simulink model "Channelizer_kernel"  (R2024a)
settings: Solver=VariableStepAuto  StartTime=0.0  StopTime=inf  RelTol=1e-3
InitFcn:
  | init
  | init_kernel
values from neighbouring files (symbols this model uses):
  N = 2*1024    (= 2048)    [hil.m]    (also in init.m = 256)
undefined symbols (not defined in the file or in its folder): ch0, ch1, ch10, ch11, ch12, ch13, ch14, ch15, ch2, ch3, ch4, ch5, ch6, ch7, ch8, ch9, S, vsva2197, xcvc1902
libraries: aieBasic x56, aieUtilities x39, hlsBasic x3, dspindex x2, vmcUtilities x1, commchan3 x1, commrflib2 x1, commfilt2 x1, commrandsrc3 x1, commdigbbndam3 x1
(part 2 of 3)

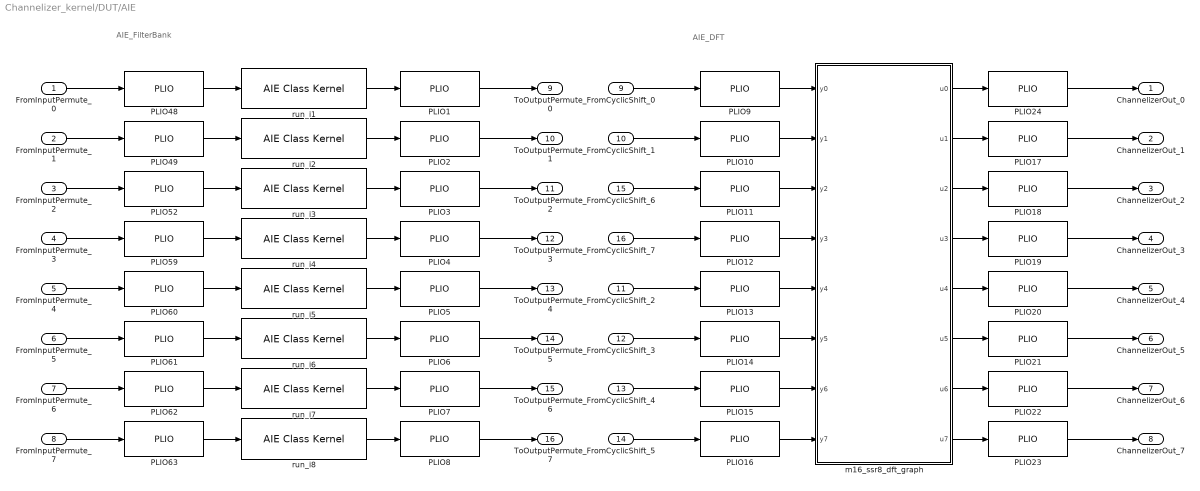
== system Channelizer_kernel/DUT/AIE ==
  note: AIE_DFT
  note: AIE_FilterBank
  FromInputPermute_0 : Inport
  FromInputPermute_1 : Inport  Port=2
  FromInputPermute_2 : Inport  Port=3
  FromInputPermute_3 : Inport  Port=4
  FromInputPermute_4 : Inport  Port=5
  FromInputPermute_5 : Inport  Port=6
  FromInputPermute_6 : Inport  Port=7
  FromInputPermute_7 : Inport  Port=8
  FromCyclicShift_0 : Inport  Port=9
  FromCyclicShift_1 : Inport  Port=10
  FromCyclicShift_2 : Inport  Port=11
  FromCyclicShift_3 : Inport  Port=12
  FromCyclicShift_4 : Inport  Port=13
  FromCyclicShift_5 : Inport  Port=14
  FromCyclicShift_6 : Inport  Port=15
  FromCyclicShift_7 : Inport  Port=16
  PLIO{1..24,48..49,52,59..63} (32 alike) : aieBasic/PLIO  PlioWidth=64  PlioFreqSpec=on  PlioFreq=625  ColLocation=0  channel=0  blockJsonConstraints=[]  deprecateConstraints=0
  m16_ssr8_dft_graph : Subsystem
  run_i1 : aieBasic/AIE Class Kernel  KernelAllAttrs=|  PortNames={'sig_i'; 'sig_o'}  PortSerializedTypes={'{Q2{P{Tinput_stream{1{t{Scint16}}}}}}'; '{Q2{P{Toutput_stream{1{t{Scint16}}}}}}'}  PortWindowSizes={0.000000000000000000e+00; 0.000000000000000000e+00}  PortWindowMargins={0.000000000000000000e+00; 0.000000000000000000e+00}  PortSynchronicities={'auto', 'auto'}  PortSignalSizes={0.000000000000000000e+00; 8.192000000000000000e+03}  ClassTemplateSpecKind=implicit  ClassTemplateParamNames={'pattern'; 'NSAMP'}  ClassTemplateParamKinds={'nontype'; 'nontype'}  ClassTemplateParamTypes={'unsigned int'; 'unsigned int'}  ClassTemplateParamValues={'0', '8192'}  ClassCtorParamNames={'taps0_i'; 'taps1_i'}  ClassCtorParamSerializedTypes={'{R{C{Bi16}64}}'; '{R{C{Bi16}64}}'}  ClassCtorParamValues={'[0;2;-4;6;-13;54;-178;1985;-20;88;-287;1822;-22;100;-326;1570;2042;6;-4;2;259;-80;23;-8;569;-166;49;-9;911;-248;74;-14;-19;93;-307;1256;-14;74;-248;911;-9;49;-166;569;-8;23;-80;259;1256;-307;93;-19;1570;-326;100;-22;1822;-287;88;-20;1985;-178;54;-13]', '[6;12;-40;124;-6;28;-95;2027;-17;74;-241;1916;-22;97;-314;1706;2027;-95;28;-6;124;-40;12;6;408;-123;36;-8;737;-209;62;-12;-21;99;-322;1419;-17;85;-281;1085;-12;62;-209;737;-8;36;-123;408;1085;-281;85;-17;1419;-322;99;-21;1706;-314;97;-22;1916;-241;74;-17]'}  ClassIndex=1  ClassCtorIndex=1  ClassTabVisible=on  ClassTemplateParamsVisible=on  ClassCtorDeclVisible=on  ClassCtorParamsVisible=on  FunctionTabVisible=on  FunctionDecl=|  PortAttrs={ 'input', 'sig_i', 'input_stream_cint16 * restrict', '', '', '', ''; 'output', 'sig_o', 'output_stream_cint16 * restrict', '', '', '', '4*N' }  PortAttrsEnables={'off', 'off', 'off', 'off', 'off', 'off', 'off';'off', 'off', 'off', 'off', 'off', 'off', 'on'}  SampleTime=-1  ClassDeclTypeOptions=C[1 1]@t74@template < unsigned int pattern, unsigned int NSAMP > class polyphase_fir;  ClassDecl=template < unsigned int pattern, unsigned int NSAMP > class polyphase_fir;  ClassTemplateParams={ 'pattern', 'unsigned int', '0'; 'NSAMP', 'unsigned int', '4*N' }  ClassTemplateParamsEnables={'off', 'off', 'on';'off', 'off', 'on'}  ClassCtorDeclTypeOptions=C[1 1]@t69@polyphase_fir(int16 ( & taps0_i ) [ 64 ], int16 ( & taps1_i ) [ 64 ])  ClassCtorDecl=polyphase_fir(int16 ( & taps0_i ) [ 64 ], int16 ( & taps1_i ) [ 64 ])  ClassCtorParams={ 'taps0_i', 'int16 ( &) [ 64 ]', 'tile0_tapsA'; 'taps1_i', 'int16 ( &) [ 64 ]', 'tile0_tapsB' }  KernelHeaderFile=aie/polyphase_fir.h  KernelClassName=polyphase_fir  KernelFunction=run_i  KernelSourceFile=aie/polyphase_fir.cpp  KernelSearchPaths={}  PreProcOptions={}  blockJsonConstraints=[]
      KernelAllAttrs=|
      | s[12;12;9;9;19;14;21;23;21;23;24;21;15;17;12;24;26;26;26;27;28;9;21;23;23;23;24;25;14;19;19;29]@FunctionNameDeclFileNamePortNamesPortTypesPortSerializedTypesPortDirectionsPortWindowSizeEnablesPortWindowMarginEnablesPortBufferSizeEnablesPortBufferMarginEnablesPortSynchronicityEnablesPortSignalSizeEnablesPortBufferSizesPortBufferMarginsFunctionDeclFunctionTemplateSpecKindFunctionTemplateParamNamesFunctionTemplateParamKindsFunctionTemplateParamTypesFunctionTemplateParamValuesFunctionTemplateParamEnablesClassDeclClassTemplateSpecKindClassTemplateParamNamesClassTemplateParamKindsClassTemplateParamTypesClassTemplateParamValuesClassTemplateParamEnablesClassCtorDeclsClassCtorParamNamesClassCtorParamTypesClassCtorParamSerializedTypes[1 1]@C[32 1]@t5@run_it25@../../aie/polyphase_fir.hC[2 1]@t5@sig_it5@sig_oC[2 1]@t30@input_stream_cint16 * restrictt31@output_stream_cint16 * restrictC[2 1]@t37@{Q2{P{Tinput_stream{1{t{Scint16}}}}}}t38@{Q2{P{Toutput_stream{1{t{Scint16}}}}}}C[2 1]@t5@inputt6@outputC[2 1]@l0@l0@C[2 1]@l0@l0@C[2 1]@l0@l0@C[2 1]@l0@l0@C[2 1]@l0@l0@C[2 1]@l0@l1@C[2 1]@nnC[2 1]@nnt158@template < unsigned int pattern, unsigned int NSAMP > 
      | void polyphase_fir::
      | run_i(input_stream_cint16 * restrict sig_i, output_stream_cint16 * restrict sig_o)t4@nonee[0 1]@e[0 1]@e[0 1]@e[0 1]@e[0 1]@t74@template < unsigned int pattern, unsigned int NSAMP > class polyphase_fir;t8@implicitC[2 1]@t7@patternt5@NSAMPC[2 1]@t7@nontypet7@nontypeC[2 1]@t12@unsigned intt12@unsigned intC[2 1]@nnC[2 1]@l1@l1@C[1 1]@t69@polyphase_fir(int16 ( & taps0_i ) [ 64 ], int16 ( & taps1_i ) [ 64 ])C[1 1]@C[2 1]@t7@taps0_it7@taps1_iC[1 1]@C[2 1]@t17@int16 ( &) [ 64 ]t17@int16 ( &) [ 64 ]C[1 1]@C[2 1]@t14@{R{C{Bi16}64}}t14@{R{C{Bi16}64}}
      FunctionDecl=|
      | template < unsigned int pattern, unsigned int NSAMP > 
      | void polyphase_fir::
      | run_i(input_stream_cint16 * restrict sig_i, output_stream_cint16 * restrict sig_o)
  run_i2 : aieBasic/AIE Class Kernel  KernelAllAttrs=|  PortNames={'sig_i'; 'sig_o'}  PortSerializedTypes={'{Q2{P{Tinput_stream{1{t{Scint16}}}}}}'; '{Q2{P{Toutput_stream{1{t{Scint16}}}}}}'}  PortWindowSizes={0.000000000000000000e+00; 0.000000000000000000e+00}  PortWindowMargins={0.000000000000000000e+00; 0.000000000000000000e+00}  PortSynchronicities={'auto', 'auto'}  PortSignalSizes={0.000000000000000000e+00; 8.192000000000000000e+03}  ClassTemplateSpecKind=implicit  ClassTemplateParamNames={'pattern'; 'NSAMP'}  ClassTemplateParamKinds={'nontype'; 'nontype'}  ClassTemplateParamTypes={'unsigned int'; 'unsigned int'}  ClassTemplateParamValues={'1', '8192'}  ClassCtorParamNames={'taps0_i'; 'taps1_i'}  ClassCtorParamSerializedTypes={'{R{C{Bi16}64}}'; '{R{C{Bi16}64}}'}  ClassCtorParamValues={'[-8;23;-80;259;0;2;-4;6;-13;54;-178;1985;-20;88;-287;1822;1985;-178;54;-13;2042;6;-4;2;259;-80;23;-8;569;-166;49;-9;-22;100;-326;1570;-19;93;-307;1256;-14;74;-248;911;-9;49;-166;569;911;-248;74;-14;1256;-307;93;-19;1570;-326;100;-22;1822;-287;88;-20]', '[-8;36;-123;408;6;12;-40;124;-6;28;-95;2027;-17;74;-241;1916;1916;-241;74;-17;2027;-95;28;-6;124;-40;12;6;408;-123;36;-8;-22;97;-314;1706;-21;99;-322;1419;-17;85;-281;1085;-12;62;-209;737;737;-209;62;-12;1085;-281;85;-17;1419;-322;99;-21;1706;-314;97;-22]'}  ClassIndex=1  ClassCtorIndex=1  ClassTabVisible=on  ClassTemplateParamsVisible=on  ClassCtorDeclVisible=on  ClassCtorParamsVisible=on  FunctionTabVisible=on  FunctionDecl=|  PortAttrs={ 'input', 'sig_i', 'input_stream_cint16 * restrict', '', '', '', ''; 'output', 'sig_o', 'output_stream_cint16 * restrict', '', '', '', '4*N' }  PortAttrsEnables={'off', 'off', 'off', 'off', 'off', 'off', 'off';'off', 'off', 'off', 'off', 'off', 'off', 'on'}  SampleTime=-1  ClassDeclTypeOptions=C[1 1]@t74@template < unsigned int pattern, unsigned int NSAMP > class polyphase_fir;  ClassDecl=template < unsigned int pattern, unsigned int NSAMP > class polyphase_fir;  ClassTemplateParams={ 'pattern', 'unsigned int', '1'; 'NSAMP', 'unsigned int', '4*N' }  ClassTemplateParamsEnables={'off', 'off', 'on';'off', 'off', 'on'}  ClassCtorDeclTypeOptions=C[1 1]@t69@polyphase_fir(int16 ( & taps0_i ) [ 64 ], int16 ( & taps1_i ) [ 64 ])  ClassCtorDecl=polyphase_fir(int16 ( & taps0_i ) [ 64 ], int16 ( & taps1_i ) [ 64 ])  ClassCtorParams={ 'taps0_i', 'int16 ( &) [ 64 ]', 'tile1_tapsA'; 'taps1_i', 'int16 ( &) [ 64 ]', 'tile1_tapsB' }  KernelHeaderFile=aie/polyphase_fir.h  KernelClassName=polyphase_fir  KernelFunction=run_i  KernelSourceFile=aie/polyphase_fir.cpp  KernelSearchPaths={}  PreProcOptions={}  blockJsonConstraints=[]
      KernelAllAttrs=|
      | s[12;12;9;9;19;14;21;23;21;23;24;21;15;17;12;24;26;26;26;27;28;9;21;23;23;23;24;25;14;19;19;29]@FunctionNameDeclFileNamePortNamesPortTypesPortSerializedTypesPortDirectionsPortWindowSizeEnablesPortWindowMarginEnablesPortBufferSizeEnablesPortBufferMarginEnablesPortSynchronicityEnablesPortSignalSizeEnablesPortBufferSizesPortBufferMarginsFunctionDeclFunctionTemplateSpecKindFunctionTemplateParamNamesFunctionTemplateParamKindsFunctionTemplateParamTypesFunctionTemplateParamValuesFunctionTemplateParamEnablesClassDeclClassTemplateSpecKindClassTemplateParamNamesClassTemplateParamKindsClassTemplateParamTypesClassTemplateParamValuesClassTemplateParamEnablesClassCtorDeclsClassCtorParamNamesClassCtorParamTypesClassCtorParamSerializedTypes[1 1]@C[32 1]@t5@run_it25@../../aie/polyphase_fir.hC[2 1]@t5@sig_it5@sig_oC[2 1]@t30@input_stream_cint16 * restrictt31@output_stream_cint16 * restrictC[2 1]@t37@{Q2{P{Tinput_stream{1{t{Scint16}}}}}}t38@{Q2{P{Toutput_stream{1{t{Scint16}}}}}}C[2 1]@t5@inputt6@outputC[2 1]@l0@l0@C[2 1]@l0@l0@C[2 1]@l0@l0@C[2 1]@l0@l0@C[2 1]@l0@l0@C[2 1]@l0@l1@C[2 1]@nnC[2 1]@nnt158@template < unsigned int pattern, unsigned int NSAMP > 
      | void polyphase_fir::
      | run_i(input_stream_cint16 * restrict sig_i, output_stream_cint16 * restrict sig_o)t4@nonee[0 1]@e[0 1]@e[0 1]@e[0 1]@e[0 1]@t74@template < unsigned int pattern, unsigned int NSAMP > class polyphase_fir;t8@implicitC[2 1]@t7@patternt5@NSAMPC[2 1]@t7@nontypet7@nontypeC[2 1]@t12@unsigned intt12@unsigned intC[2 1]@nnC[2 1]@l1@l1@C[1 1]@t69@polyphase_fir(int16 ( & taps0_i ) [ 64 ], int16 ( & taps1_i ) [ 64 ])C[1 1]@C[2 1]@t7@taps0_it7@taps1_iC[1 1]@C[2 1]@t17@int16 ( &) [ 64 ]t17@int16 ( &) [ 64 ]C[1 1]@C[2 1]@t14@{R{C{Bi16}64}}t14@{R{C{Bi16}64}}
      FunctionDecl=|
      | template < unsigned int pattern, unsigned int NSAMP > 
      | void polyphase_fir::
      | run_i(input_stream_cint16 * restrict sig_i, output_stream_cint16 * restrict sig_o)
  run_i3 : aieBasic/AIE Class Kernel  KernelAllAttrs=|  PortNames={'sig_i'; 'sig_o'}  PortSerializedTypes={'{Q2{P{Tinput_stream{1{t{Scint16}}}}}}'; '{Q2{P{Toutput_stream{1{t{Scint16}}}}}}'}  PortWindowSizes={0.000000000000000000e+00; 0.000000000000000000e+00}  PortWindowMargins={0.000000000000000000e+00; 0.000000000000000000e+00}  PortSynchronicities={'auto', 'auto'}  PortSignalSizes={0.000000000000000000e+00; 8.192000000000000000e+03}  ClassTemplateSpecKind=implicit  ClassTemplateParamNames={'pattern'; 'NSAMP'}  ClassTemplateParamKinds={'nontype'; 'nontype'}  ClassTemplateParamTypes={'unsigned int'; 'unsigned int'}  ClassTemplateParamValues={'2', '8192'}  ClassCtorParamNames={'taps0_i'; 'taps1_i'}  ClassCtorParamSerializedTypes={'{R{C{Bi16}64}}'; '{R{C{Bi16}64}}'}  ClassCtorParamValues={'[-9;49;-166;569;-8;23;-80;259;0;2;-4;6;-13;54;-178;1985;1822;-287;88;-20;1985;-178;54;-13;2042;6;-4;2;259;-80;23;-8;-20;88;-287;1822;-22;100;-326;1570;-19;93;-307;1256;-14;74;-248;911;569;-166;49;-9;911;-248;74;-14;1256;-307;93;-19;1570;-326;100;-22]', '[-12;62;-209;737;-8;36;-123;408;6;12;-40;124;-6;28;-95;2027;1706;-314;97;-22;1916;-241;74;-17;2027;-95;28;-6;124;-40;12;6;-17;74;-241;1916;-22;97;-314;1706;-21;99;-322;1419;-17;85;-281;1085;408;-123;36;-8;737;-209;62;-12;1085;-281;85;-17;1419;-322;99;-21]'}  ClassIndex=1  ClassCtorIndex=1  ClassTabVisible=on  ClassTemplateParamsVisible=on  ClassCtorDeclVisible=on  ClassCtorParamsVisible=on  FunctionTabVisible=on  FunctionDecl=|  PortAttrs={ 'input', 'sig_i', 'input_stream_cint16 * restrict', '', '', '', ''; 'output', 'sig_o', 'output_stream_cint16 * restrict', '', '', '', '4*N' }  PortAttrsEnables={'off', 'off', 'off', 'off', 'off', 'off', 'off';'off', 'off', 'off', 'off', 'off', 'off', 'on'}  SampleTime=-1  ClassDeclTypeOptions=C[1 1]@t74@template < unsigned int pattern, unsigned int NSAMP > class polyphase_fir;  ClassDecl=template < unsigned int pattern, unsigned int NSAMP > class polyphase_fir;  ClassTemplateParams={ 'pattern', 'unsigned int', '2'; 'NSAMP', 'unsigned int', '4*N' }  ClassTemplateParamsEnables={'off', 'off', 'on';'off', 'off', 'on'}  ClassCtorDeclTypeOptions=C[1 1]@t69@polyphase_fir(int16 ( & taps0_i ) [ 64 ], int16 ( & taps1_i ) [ 64 ])  ClassCtorDecl=polyphase_fir(int16 ( & taps0_i ) [ 64 ], int16 ( & taps1_i ) [ 64 ])  ClassCtorParams={ 'taps0_i', 'int16 ( &) [ 64 ]', 'tile2_tapsA'; 'taps1_i', 'int16 ( &) [ 64 ]', 'tile2_tapsB' }  KernelHeaderFile=aie/polyphase_fir.h  KernelClassName=polyphase_fir  KernelFunction=run_i  KernelSourceFile=aie/polyphase_fir.cpp  KernelSearchPaths={}  PreProcOptions={}  blockJsonConstraints=[]
      KernelAllAttrs=|
      | s[12;12;9;9;19;14;21;23;21;23;24;21;15;17;12;24;26;26;26;27;28;9;21;23;23;23;24;25;14;19;19;29]@FunctionNameDeclFileNamePortNamesPortTypesPortSerializedTypesPortDirectionsPortWindowSizeEnablesPortWindowMarginEnablesPortBufferSizeEnablesPortBufferMarginEnablesPortSynchronicityEnablesPortSignalSizeEnablesPortBufferSizesPortBufferMarginsFunctionDeclFunctionTemplateSpecKindFunctionTemplateParamNamesFunctionTemplateParamKindsFunctionTemplateParamTypesFunctionTemplateParamValuesFunctionTemplateParamEnablesClassDeclClassTemplateSpecKindClassTemplateParamNamesClassTemplateParamKindsClassTemplateParamTypesClassTemplateParamValuesClassTemplateParamEnablesClassCtorDeclsClassCtorParamNamesClassCtorParamTypesClassCtorParamSerializedTypes[1 1]@C[32 1]@t5@run_it25@../../aie/polyphase_fir.hC[2 1]@t5@sig_it5@sig_oC[2 1]@t30@input_stream_cint16 * restrictt31@output_stream_cint16 * restrictC[2 1]@t37@{Q2{P{Tinput_stream{1{t{Scint16}}}}}}t38@{Q2{P{Toutput_stream{1{t{Scint16}}}}}}C[2 1]@t5@inputt6@outputC[2 1]@l0@l0@C[2 1]@l0@l0@C[2 1]@l0@l0@C[2 1]@l0@l0@C[2 1]@l0@l0@C[2 1]@l0@l1@C[2 1]@nnC[2 1]@nnt158@template < unsigned int pattern, unsigned int NSAMP > 
      | void polyphase_fir::
      | run_i(input_stream_cint16 * restrict sig_i, output_stream_cint16 * restrict sig_o)t4@nonee[0 1]@e[0 1]@e[0 1]@e[0 1]@e[0 1]@t74@template < unsigned int pattern, unsigned int NSAMP > class polyphase_fir;t8@implicitC[2 1]@t7@patternt5@NSAMPC[2 1]@t7@nontypet7@nontypeC[2 1]@t12@unsigned intt12@unsigned intC[2 1]@nnC[2 1]@l1@l1@C[1 1]@t69@polyphase_fir(int16 ( & taps0_i ) [ 64 ], int16 ( & taps1_i ) [ 64 ])C[1 1]@C[2 1]@t7@taps0_it7@taps1_iC[1 1]@C[2 1]@t17@int16 ( &) [ 64 ]t17@int16 ( &) [ 64 ]C[1 1]@C[2 1]@t14@{R{C{Bi16}64}}t14@{R{C{Bi16}64}}
      FunctionDecl=|
      | template < unsigned int pattern, unsigned int NSAMP > 
      | void polyphase_fir::
      | run_i(input_stream_cint16 * restrict sig_i, output_stream_cint16 * restrict sig_o)
  run_i4 : aieBasic/AIE Class Kernel  KernelAllAttrs=|  PortNames={'sig_i'; 'sig_o'}  PortSerializedTypes={'{Q2{P{Tinput_stream{1{t{Scint16}}}}}}'; '{Q2{P{Toutput_stream{1{t{Scint16}}}}}}'}  PortWindowSizes={0.000000000000000000e+00; 0.000000000000000000e+00}  PortWindowMargins={0.000000000000000000e+00; 0.000000000000000000e+00}  PortSynchronicities={'auto', 'auto'}  PortSignalSizes={0.000000000000000000e+00; 8.192000000000000000e+03}  ClassTemplateSpecKind=implicit  ClassTemplateParamNames={'pattern'; 'NSAMP'}  ClassTemplateParamKinds={'nontype'; 'nontype'}  ClassTemplateParamTypes={'unsigned int'; 'unsigned int'}  ClassTemplateParamValues={'3', '8192'}  ClassCtorParamNames={'taps0_i'; 'taps1_i'}  ClassCtorParamSerializedTypes={'{R{C{Bi16}64}}'; '{R{C{Bi16}64}}'}  ClassCtorParamValues={'[-14;74;-248;911;-9;49;-166;569;-8;23;-80;259;0;2;-4;6;1570;-326;100;-22;1822;-287;88;-20;1985;-178;54;-13;2042;6;-4;2;-13;54;-178;1985;-20;88;-287;1822;-22;100;-326;1570;-19;93;-307;1256;259;-80;23;-8;569;-166;49;-9;911;-248;74;-14;1256;-307;93;-19]', '[-17;85;-281;1085;-12;62;-209;737;-8;36;-123;408;6;12;-40;124;1419;-322;99;-21;1706;-314;97;-22;1916;-241;74;-17;2027;-95;28;-6;-6;28;-95;2027;-17;74;-241;1916;-22;97;-314;1706;-21;99;-322;1419;124;-40;12;6;408;-123;36;-8;737;-209;62;-12;1085;-281;85;-17]'}  ClassIndex=1  ClassCtorIndex=1  ClassTabVisible=on  ClassTemplateParamsVisible=on  ClassCtorDeclVisible=on  ClassCtorParamsVisible=on  FunctionTabVisible=on  FunctionDecl=|  PortAttrs={ 'input', 'sig_i', 'input_stream_cint16 * restrict', '', '', '', ''; 'output', 'sig_o', 'output_stream_cint16 * restrict', '', '', '', '4*N' }  PortAttrsEnables={'off', 'off', 'off', 'off', 'off', 'off', 'off';'off', 'off', 'off', 'off', 'off', 'off', 'on'}  SampleTime=-1  ClassDeclTypeOptions=C[1 1]@t74@template < unsigned int pattern, unsigned int NSAMP > class polyphase_fir;  ClassDecl=template < unsigned int pattern, unsigned int NSAMP > class polyphase_fir;  ClassTemplateParams={ 'pattern', 'unsigned int', '3'; 'NSAMP', 'unsigned int', '4*N' }  ClassTemplateParamsEnables={'off', 'off', 'on';'off', 'off', 'on'}  ClassCtorDeclTypeOptions=C[1 1]@t69@polyphase_fir(int16 ( & taps0_i ) [ 64 ], int16 ( & taps1_i ) [ 64 ])  ClassCtorDecl=polyphase_fir(int16 ( & taps0_i ) [ 64 ], int16 ( & taps1_i ) [ 64 ])  ClassCtorParams={ 'taps0_i', 'int16 ( &) [ 64 ]', 'tile3_tapsA'; 'taps1_i', 'int16 ( &) [ 64 ]', 'tile3_tapsB' }  KernelHeaderFile=aie/polyphase_fir.h  KernelClassName=polyphase_fir  KernelFunction=run_i  KernelSourceFile=aie/polyphase_fir.cpp  KernelSearchPaths={}  PreProcOptions={}  blockJsonConstraints=[]
      KernelAllAttrs=|
      | s[12;12;9;9;19;14;21;23;21;23;24;21;15;17;12;24;26;26;26;27;28;9;21;23;23;23;24;25;14;19;19;29]@FunctionNameDeclFileNamePortNamesPortTypesPortSerializedTypesPortDirectionsPortWindowSizeEnablesPortWindowMarginEnablesPortBufferSizeEnablesPortBufferMarginEnablesPortSynchronicityEnablesPortSignalSizeEnablesPortBufferSizesPortBufferMarginsFunctionDeclFunctionTemplateSpecKindFunctionTemplateParamNamesFunctionTemplateParamKindsFunctionTemplateParamTypesFunctionTemplateParamValuesFunctionTemplateParamEnablesClassDeclClassTemplateSpecKindClassTemplateParamNamesClassTemplateParamKindsClassTemplateParamTypesClassTemplateParamValuesClassTemplateParamEnablesClassCtorDeclsClassCtorParamNamesClassCtorParamTypesClassCtorParamSerializedTypes[1 1]@C[32 1]@t5@run_it25@../../aie/polyphase_fir.hC[2 1]@t5@sig_it5@sig_oC[2 1]@t30@input_stream_cint16 * restrictt31@output_stream_cint16 * restrictC[2 1]@t37@{Q2{P{Tinput_stream{1{t{Scint16}}}}}}t38@{Q2{P{Toutput_stream{1{t{Scint16}}}}}}C[2 1]@t5@inputt6@outputC[2 1]@l0@l0@C[2 1]@l0@l0@C[2 1]@l0@l0@C[2 1]@l0@l0@C[2 1]@l0@l0@C[2 1]@l0@l1@C[2 1]@nnC[2 1]@nnt158@template < unsigned int pattern, unsigned int NSAMP > 
      | void polyphase_fir::
      | run_i(input_stream_cint16 * restrict sig_i, output_stream_cint16 * restrict sig_o)t4@nonee[0 1]@e[0 1]@e[0 1]@e[0 1]@e[0 1]@t74@template < unsigned int pattern, unsigned int NSAMP > class polyphase_fir;t8@implicitC[2 1]@t7@patternt5@NSAMPC[2 1]@t7@nontypet7@nontypeC[2 1]@t12@unsigned intt12@unsigned intC[2 1]@nnC[2 1]@l1@l1@C[1 1]@t69@polyphase_fir(int16 ( & taps0_i ) [ 64 ], int16 ( & taps1_i ) [ 64 ])C[1 1]@C[2 1]@t7@taps0_it7@taps1_iC[1 1]@C[2 1]@t17@int16 ( &) [ 64 ]t17@int16 ( &) [ 64 ]C[1 1]@C[2 1]@t14@{R{C{Bi16}64}}t14@{R{C{Bi16}64}}
      FunctionDecl=|
      | template < unsigned int pattern, unsigned int NSAMP > 
      | void polyphase_fir::
      | run_i(input_stream_cint16 * restrict sig_i, output_stream_cint16 * restrict sig_o)
  run_i5 : aieBasic/AIE Class Kernel  KernelAllAttrs=|  PortNames={'sig_i'; 'sig_o'}  PortSerializedTypes={'{Q2{P{Tinput_stream{1{t{Scint16}}}}}}'; '{Q2{P{Toutput_stream{1{t{Scint16}}}}}}'}  PortWindowSizes={0.000000000000000000e+00; 0.000000000000000000e+00}  PortWindowMargins={0.000000000000000000e+00; 0.000000000000000000e+00}  PortSynchronicities={'auto', 'auto'}  PortSignalSizes={0.000000000000000000e+00; 8.192000000000000000e+03}  ClassTemplateSpecKind=implicit  ClassTemplateParamNames={'pattern'; 'NSAMP'}  ClassTemplateParamKinds={'nontype'; 'nontype'}  ClassTemplateParamTypes={'unsigned int'; 'unsigned int'}  ClassTemplateParamValues={'4', '8192'}  ClassCtorParamNames={'taps0_i'; 'taps1_i'}  ClassCtorParamSerializedTypes={'{R{C{Bi16}64}}'; '{R{C{Bi16}64}}'}  ClassCtorParamValues={'[-19;93;-307;1256;-14;74;-248;911;-9;49;-166;569;-8;23;-80;259;1256;-307;93;-19;1570;-326;100;-22;1822;-287;88;-20;1985;-178;54;-13;0;2;-4;6;-13;54;-178;1985;-20;88;-287;1822;-22;100;-326;1570;2042;6;-4;2;259;-80;23;-8;569;-166;49;-9;911;-248;74;-14]', '[-21;99;-322;1419;-17;85;-281;1085;-12;62;-209;737;-8;36;-123;408;1085;-281;85;-17;1419;-322;99;-21;1706;-314;97;-22;1916;-241;74;-17;6;12;-40;124;-6;28;-95;2027;-17;74;-241;1916;-22;97;-314;1706;2027;-95;28;-6;124;-40;12;6;408;-123;36;-8;737;-209;62;-12]'}  ClassIndex=1  ClassCtorIndex=1  ClassTabVisible=on  ClassTemplateParamsVisible=on  ClassCtorDeclVisible=on  ClassCtorParamsVisible=on  FunctionTabVisible=on  FunctionDecl=|  PortAttrs={ 'input', 'sig_i', 'input_stream_cint16 * restrict', '', '', '', ''; 'output', 'sig_o', 'output_stream_cint16 * restrict', '', '', '', '4*N' }  PortAttrsEnables={'off', 'off', 'off', 'off', 'off', 'off', 'off';'off', 'off', 'off', 'off', 'off', 'off', 'on'}  SampleTime=-1  ClassDeclTypeOptions=C[1 1]@t74@template < unsigned int pattern, unsigned int NSAMP > class polyphase_fir;  ClassDecl=template < unsigned int pattern, unsigned int NSAMP > class polyphase_fir;  ClassTemplateParams={ 'pattern', 'unsigned int', '4'; 'NSAMP', 'unsigned int', '4*N' }  ClassTemplateParamsEnables={'off', 'off', 'on';'off', 'off', 'on'}  ClassCtorDeclTypeOptions=C[1 1]@t69@polyphase_fir(int16 ( & taps0_i ) [ 64 ], int16 ( & taps1_i ) [ 64 ])  ClassCtorDecl=polyphase_fir(int16 ( & taps0_i ) [ 64 ], int16 ( & taps1_i ) [ 64 ])  ClassCtorParams={ 'taps0_i', 'int16 ( &) [ 64 ]', 'tile4_tapsA'; 'taps1_i', 'int16 ( &) [ 64 ]', 'tile4_tapsB' }  KernelHeaderFile=aie/polyphase_fir.h  KernelClassName=polyphase_fir  KernelFunction=run_i  KernelSourceFile=aie/polyphase_fir.cpp  KernelSearchPaths={}  PreProcOptions={}  blockJsonConstraints=[]
      KernelAllAttrs=|
      | s[12;12;9;9;19;14;21;23;21;23;24;21;15;17;12;24;26;26;26;27;28;9;21;23;23;23;24;25;14;19;19;29]@FunctionNameDeclFileNamePortNamesPortTypesPortSerializedTypesPortDirectionsPortWindowSizeEnablesPortWindowMarginEnablesPortBufferSizeEnablesPortBufferMarginEnablesPortSynchronicityEnablesPortSignalSizeEnablesPortBufferSizesPortBufferMarginsFunctionDeclFunctionTemplateSpecKindFunctionTemplateParamNamesFunctionTemplateParamKindsFunctionTemplateParamTypesFunctionTemplateParamValuesFunctionTemplateParamEnablesClassDeclClassTemplateSpecKindClassTemplateParamNamesClassTemplateParamKindsClassTemplateParamTypesClassTemplateParamValuesClassTemplateParamEnablesClassCtorDeclsClassCtorParamNamesClassCtorParamTypesClassCtorParamSerializedTypes[1 1]@C[32 1]@t5@run_it25@../../aie/polyphase_fir.hC[2 1]@t5@sig_it5@sig_oC[2 1]@t30@input_stream_cint16 * restrictt31@output_stream_cint16 * restrictC[2 1]@t37@{Q2{P{Tinput_stream{1{t{Scint16}}}}}}t38@{Q2{P{Toutput_stream{1{t{Scint16}}}}}}C[2 1]@t5@inputt6@outputC[2 1]@l0@l0@C[2 1]@l0@l0@C[2 1]@l0@l0@C[2 1]@l0@l0@C[2 1]@l0@l0@C[2 1]@l0@l1@C[2 1]@nnC[2 1]@nnt158@template < unsigned int pattern, unsigned int NSAMP > 
      | void polyphase_fir::
      | run_i(input_stream_cint16 * restrict sig_i, output_stream_cint16 * restrict sig_o)t4@nonee[0 1]@e[0 1]@e[0 1]@e[0 1]@e[0 1]@t74@template < unsigned int pattern, unsigned int NSAMP > class polyphase_fir;t8@implicitC[2 1]@t7@patternt5@NSAMPC[2 1]@t7@nontypet7@nontypeC[2 1]@t12@unsigned intt12@unsigned intC[2 1]@nnC[2 1]@l1@l1@C[1 1]@t69@polyphase_fir(int16 ( & taps0_i ) [ 64 ], int16 ( & taps1_i ) [ 64 ])C[1 1]@C[2 1]@t7@taps0_it7@taps1_iC[1 1]@C[2 1]@t17@int16 ( &) [ 64 ]t17@int16 ( &) [ 64 ]C[1 1]@C[2 1]@t14@{R{C{Bi16}64}}t14@{R{C{Bi16}64}}
      FunctionDecl=|
      | template < unsigned int pattern, unsigned int NSAMP > 
      | void polyphase_fir::
      | run_i(input_stream_cint16 * restrict sig_i, output_stream_cint16 * restrict sig_o)
  run_i6 : aieBasic/AIE Class Kernel  KernelAllAttrs=|  PortNames={'sig_i'; 'sig_o'}  PortSerializedTypes={'{Q2{P{Tinput_stream{1{t{Scint16}}}}}}'; '{Q2{P{Toutput_stream{1{t{Scint16}}}}}}'}  PortWindowSizes={0.000000000000000000e+00; 0.000000000000000000e+00}  PortWindowMargins={0.000000000000000000e+00; 0.000000000000000000e+00}  PortSynchronicities={'auto', 'auto'}  PortSignalSizes={0.000000000000000000e+00; 8.192000000000000000e+03}  ClassTemplateSpecKind=implicit  ClassTemplateParamNames={'pattern'; 'NSAMP'}  ClassTemplateParamKinds={'nontype'; 'nontype'}  ClassTemplateParamTypes={'unsigned int'; 'unsigned int'}  ClassTemplateParamValues={'5', '8192'}  ClassCtorParamNames={'taps0_i'; 'taps1_i'}  ClassCtorParamSerializedTypes={'{R{C{Bi16}64}}'; '{R{C{Bi16}64}}'}  ClassCtorParamValues={'[-22;100;-326;1570;-19;93;-307;1256;-14;74;-248;911;-9;49;-166;569;911;-248;74;-14;1256;-307;93;-19;1570;-326;100;-22;1822;-287;88;-20;-8;23;-80;259;0;2;-4;6;-13;54;-178;1985;-20;88;-287;1822;1985;-178;54;-13;2042;6;-4;2;259;-80;23;-8;569;-166;49;-9]', '[-22;97;-314;1706;-21;99;-322;1419;-17;85;-281;1085;-12;62;-209;737;737;-209;62;-12;1085;-281;85;-17;1419;-322;99;-21;1706;-314;97;-22;-8;36;-123;408;6;12;-40;124;-6;28;-95;2027;-17;74;-241;1916;1916;-241;74;-17;2027;-95;28;-6;124;-40;12;6;408;-123;36;-8]'}  ClassIndex=1  ClassCtorIndex=1  ClassTabVisible=on  ClassTemplateParamsVisible=on  ClassCtorDeclVisible=on  ClassCtorParamsVisible=on  FunctionTabVisible=on  FunctionDecl=|  PortAttrs={ 'input', 'sig_i', 'input_stream_cint16 * restrict', '', '', '', ''; 'output', 'sig_o', 'output_stream_cint16 * restrict', '', '', '', '4*N' }  PortAttrsEnables={'off', 'off', 'off', 'off', 'off', 'off', 'off';'off', 'off', 'off', 'off', 'off', 'off', 'on'}  SampleTime=-1  ClassDeclTypeOptions=C[1 1]@t74@template < unsigned int pattern, unsigned int NSAMP > class polyphase_fir;  ClassDecl=template < unsigned int pattern, unsigned int NSAMP > class polyphase_fir;  ClassTemplateParams={ 'pattern', 'unsigned int', '5'; 'NSAMP', 'unsigned int', '4*N' }  ClassTemplateParamsEnables={'off', 'off', 'on';'off', 'off', 'on'}  ClassCtorDeclTypeOptions=C[1 1]@t69@polyphase_fir(int16 ( & taps0_i ) [ 64 ], int16 ( & taps1_i ) [ 64 ])  ClassCtorDecl=polyphase_fir(int16 ( & taps0_i ) [ 64 ], int16 ( & taps1_i ) [ 64 ])  ClassCtorParams={ 'taps0_i', 'int16 ( &) [ 64 ]', 'tile5_tapsA'; 'taps1_i', 'int16 ( &) [ 64 ]', 'tile5_tapsB' }  KernelHeaderFile=aie/polyphase_fir.h  KernelClassName=polyphase_fir  KernelFunction=run_i  KernelSourceFile=aie/polyphase_fir.cpp  KernelSearchPaths={}  PreProcOptions={}  blockJsonConstraints=[]
      KernelAllAttrs=|
      | s[12;12;9;9;19;14;21;23;21;23;24;21;15;17;12;24;26;26;26;27;28;9;21;23;23;23;24;25;14;19;19;29]@FunctionNameDeclFileNamePortNamesPortTypesPortSerializedTypesPortDirectionsPortWindowSizeEnablesPortWindowMarginEnablesPortBufferSizeEnablesPortBufferMarginEnablesPortSynchronicityEnablesPortSignalSizeEnablesPortBufferSizesPortBufferMarginsFunctionDeclFunctionTemplateSpecKindFunctionTemplateParamNamesFunctionTemplateParamKindsFunctionTemplateParamTypesFunctionTemplateParamValuesFunctionTemplateParamEnablesClassDeclClassTemplateSpecKindClassTemplateParamNamesClassTemplateParamKindsClassTemplateParamTypesClassTemplateParamValuesClassTemplateParamEnablesClassCtorDeclsClassCtorParamNamesClassCtorParamTypesClassCtorParamSerializedTypes[1 1]@C[32 1]@t5@run_it25@../../aie/polyphase_fir.hC[2 1]@t5@sig_it5@sig_oC[2 1]@t30@input_stream_cint16 * restrictt31@output_stream_cint16 * restrictC[2 1]@t37@{Q2{P{Tinput_stream{1{t{Scint16}}}}}}t38@{Q2{P{Toutput_stream{1{t{Scint16}}}}}}C[2 1]@t5@inputt6@outputC[2 1]@l0@l0@C[2 1]@l0@l0@C[2 1]@l0@l0@C[2 1]@l0@l0@C[2 1]@l0@l0@C[2 1]@l0@l1@C[2 1]@nnC[2 1]@nnt158@template < unsigned int pattern, unsigned int NSAMP > 
      | void polyphase_fir::
      | run_i(input_stream_cint16 * restrict sig_i, output_stream_cint16 * restrict sig_o)t4@nonee[0 1]@e[0 1]@e[0 1]@e[0 1]@e[0 1]@t74@template < unsigned int pattern, unsigned int NSAMP > class polyphase_fir;t8@implicitC[2 1]@t7@patternt5@NSAMPC[2 1]@t7@nontypet7@nontypeC[2 1]@t12@unsigned intt12@unsigned intC[2 1]@nnC[2 1]@l1@l1@C[1 1]@t69@polyphase_fir(int16 ( & taps0_i ) [ 64 ], int16 ( & taps1_i ) [ 64 ])C[1 1]@C[2 1]@t7@taps0_it7@taps1_iC[1 1]@C[2 1]@t17@int16 ( &) [ 64 ]t17@int16 ( &) [ 64 ]C[1 1]@C[2 1]@t14@{R{C{Bi16}64}}t14@{R{C{Bi16}64}}
      FunctionDecl=|
      | template < unsigned int pattern, unsigned int NSAMP > 
      | void polyphase_fir::
      | run_i(input_stream_cint16 * restrict sig_i, output_stream_cint16 * restrict sig_o)
  run_i7 : aieBasic/AIE Class Kernel  KernelAllAttrs=|  PortNames={'sig_i'; 'sig_o'}  PortSerializedTypes={'{Q2{P{Tinput_stream{1{t{Scint16}}}}}}'; '{Q2{P{Toutput_stream{1{t{Scint16}}}}}}'}  PortWindowSizes={0.000000000000000000e+00; 0.000000000000000000e+00}  PortWindowMargins={0.000000000000000000e+00; 0.000000000000000000e+00}  PortSynchronicities={'auto', 'auto'}  PortSignalSizes={0.000000000000000000e+00; 8.192000000000000000e+03}  ClassTemplateSpecKind=implicit  ClassTemplateParamNames={'pattern'; 'NSAMP'}  ClassTemplateParamKinds={'nontype'; 'nontype'}  ClassTemplateParamTypes={'unsigned int'; 'unsigned int'}  ClassTemplateParamValues={'6', '8192'}  ClassCtorParamNames={'taps0_i'; 'taps1_i'}  ClassCtorParamSerializedTypes={'{R{C{Bi16}64}}'; '{R{C{Bi16}64}}'}  ClassCtorParamValues={'[-20;88;-287;1822;-22;100;-326;1570;-19;93;-307;1256;-14;74;-248;911;569;-166;49;-9;911;-248;74;-14;1256;-307;93;-19;1570;-326;100;-22;-9;49;-166;569;-8;23;-80;259;0;2;-4;6;-13;54;-178;1985;1822;-287;88;-20;1985;-178;54;-13;2042;6;-4;2;259;-80;23;-8]', '[-17;74;-241;1916;-22;97;-314;1706;-21;99;-322;1419;-17;85;-281;1085;408;-123;36;-8;737;-209;62;-12;1085;-281;85;-17;1419;-322;99;-21;-12;62;-209;737;-8;36;-123;408;6;12;-40;124;-6;28;-95;2027;1706;-314;97;-22;1916;-241;74;-17;2027;-95;28;-6;124;-40;12;6]'}  ClassIndex=1  ClassCtorIndex=1  ClassTabVisible=on  ClassTemplateParamsVisible=on  ClassCtorDeclVisible=on  ClassCtorParamsVisible=on  FunctionTabVisible=on  FunctionDecl=|  PortAttrs={ 'input', 'sig_i', 'input_stream_cint16 * restrict', '', '', '', ''; 'output', 'sig_o', 'output_stream_cint16 * restrict', '', '', '', '4*N' }  PortAttrsEnables={'off', 'off', 'off', 'off', 'off', 'off', 'off';'off', 'off', 'off', 'off', 'off', 'off', 'on'}  SampleTime=-1  ClassDeclTypeOptions=C[1 1]@t74@template < unsigned int pattern, unsigned int NSAMP > class polyphase_fir;  ClassDecl=template < unsigned int pattern, unsigned int NSAMP > class polyphase_fir;  ClassTemplateParams={ 'pattern', 'unsigned int', '6'; 'NSAMP', 'unsigned int', '4*N' }  ClassTemplateParamsEnables={'off', 'off', 'on';'off', 'off', 'on'}  ClassCtorDeclTypeOptions=C[1 1]@t69@polyphase_fir(int16 ( & taps0_i ) [ 64 ], int16 ( & taps1_i ) [ 64 ])  ClassCtorDecl=polyphase_fir(int16 ( & taps0_i ) [ 64 ], int16 ( & taps1_i ) [ 64 ])  ClassCtorParams={ 'taps0_i', 'int16 ( &) [ 64 ]', 'tile6_tapsA'; 'taps1_i', 'int16 ( &) [ 64 ]', 'tile6_tapsB' }  KernelHeaderFile=aie/polyphase_fir.h  KernelClassName=polyphase_fir  KernelFunction=run_i  KernelSourceFile=aie/polyphase_fir.cpp  KernelSearchPaths={}  PreProcOptions={}  blockJsonConstraints=[]
      KernelAllAttrs=|
      | s[12;12;9;9;19;14;21;23;21;23;24;21;15;17;12;24;26;26;26;27;28;9;21;23;23;23;24;25;14;19;19;29]@FunctionNameDeclFileNamePortNamesPortTypesPortSerializedTypesPortDirectionsPortWindowSizeEnablesPortWindowMarginEnablesPortBufferSizeEnablesPortBufferMarginEnablesPortSynchronicityEnablesPortSignalSizeEnablesPortBufferSizesPortBufferMarginsFunctionDeclFunctionTemplateSpecKindFunctionTemplateParamNamesFunctionTemplateParamKindsFunctionTemplateParamTypesFunctionTemplateParamValuesFunctionTemplateParamEnablesClassDeclClassTemplateSpecKindClassTemplateParamNamesClassTemplateParamKindsClassTemplateParamTypesClassTemplateParamValuesClassTemplateParamEnablesClassCtorDeclsClassCtorParamNamesClassCtorParamTypesClassCtorParamSerializedTypes[1 1]@C[32 1]@t5@run_it25@../../aie/polyphase_fir.hC[2 1]@t5@sig_it5@sig_oC[2 1]@t30@input_stream_cint16 * restrictt31@output_stream_cint16 * restrictC[2 1]@t37@{Q2{P{Tinput_stream{1{t{Scint16}}}}}}t38@{Q2{P{Toutput_stream{1{t{Scint16}}}}}}C[2 1]@t5@inputt6@outputC[2 1]@l0@l0@C[2 1]@l0@l0@C[2 1]@l0@l0@C[2 1]@l0@l0@C[2 1]@l0@l0@C[2 1]@l0@l1@C[2 1]@nnC[2 1]@nnt158@template < unsigned int pattern, unsigned int NSAMP > 
      | void polyphase_fir::
      | run_i(input_stream_cint16 * restrict sig_i, output_stream_cint16 * restrict sig_o)t4@nonee[0 1]@e[0 1]@e[0 1]@e[0 1]@e[0 1]@t74@template < unsigned int pattern, unsigned int NSAMP > class polyphase_fir;t8@implicitC[2 1]@t7@patternt5@NSAMPC[2 1]@t7@nontypet7@nontypeC[2 1]@t12@unsigned intt12@unsigned intC[2 1]@nnC[2 1]@l1@l1@C[1 1]@t69@polyphase_fir(int16 ( & taps0_i ) [ 64 ], int16 ( & taps1_i ) [ 64 ])C[1 1]@C[2 1]@t7@taps0_it7@taps1_iC[1 1]@C[2 1]@t17@int16 ( &) [ 64 ]t17@int16 ( &) [ 64 ]C[1 1]@C[2 1]@t14@{R{C{Bi16}64}}t14@{R{C{Bi16}64}}
      FunctionDecl=|
      | template < unsigned int pattern, unsigned int NSAMP > 
      | void polyphase_fir::
      | run_i(input_stream_cint16 * restrict sig_i, output_stream_cint16 * restrict sig_o)
  run_i8 : aieBasic/AIE Class Kernel  KernelAllAttrs=|  PortNames={'sig_i'; 'sig_o'}  PortSerializedTypes={'{Q2{P{Tinput_stream{1{t{Scint16}}}}}}'; '{Q2{P{Toutput_stream{1{t{Scint16}}}}}}'}  PortWindowSizes={0.000000000000000000e+00; 0.000000000000000000e+00}  PortWindowMargins={0.000000000000000000e+00; 0.000000000000000000e+00}  PortSynchronicities={'auto', 'auto'}  PortSignalSizes={0.000000000000000000e+00; 8.192000000000000000e+03}  ClassTemplateSpecKind=implicit  ClassTemplateParamNames={'pattern'; 'NSAMP'}  ClassTemplateParamKinds={'nontype'; 'nontype'}  ClassTemplateParamTypes={'unsigned int'; 'unsigned int'}  ClassTemplateParamValues={'7', '8192'}  ClassCtorParamNames={'taps0_i'; 'taps1_i'}  ClassCtorParamSerializedTypes={'{R{C{Bi16}64}}'; '{R{C{Bi16}64}}'}  ClassCtorParamValues={'[-13;54;-178;1985;-20;88;-287;1822;-22;100;-326;1570;-19;93;-307;1256;259;-80;23;-8;569;-166;49;-9;911;-248;74;-14;1256;-307;93;-19;-14;74;-248;911;-9;49;-166;569;-8;23;-80;259;0;2;-4;6;1570;-326;100;-22;1822;-287;88;-20;1985;-178;54;-13;2042;6;-4;2]', '[-6;28;-95;2027;-17;74;-241;1916;-22;97;-314;1706;-21;99;-322;1419;124;-40;12;6;408;-123;36;-8;737;-209;62;-12;1085;-281;85;-17;-17;85;-281;1085;-12;62;-209;737;-8;36;-123;408;6;12;-40;124;1419;-322;99;-21;1706;-314;97;-22;1916;-241;74;-17;2027;-95;28;-6]'}  ClassIndex=1  ClassCtorIndex=1  ClassTabVisible=on  ClassTemplateParamsVisible=on  ClassCtorDeclVisible=on  ClassCtorParamsVisible=on  FunctionTabVisible=on  FunctionDecl=|  PortAttrs={ 'input', 'sig_i', 'input_stream_cint16 * restrict', '', '', '', ''; 'output', 'sig_o', 'output_stream_cint16 * restrict', '', '', '', '4*N' }  PortAttrsEnables={'off', 'off', 'off', 'off', 'off', 'off', 'off';'off', 'off', 'off', 'off', 'off', 'off', 'on'}  SampleTime=-1  ClassDeclTypeOptions=C[1 1]@t74@template < unsigned int pattern, unsigned int NSAMP > class polyphase_fir;  ClassDecl=template < unsigned int pattern, unsigned int NSAMP > class polyphase_fir;  ClassTemplateParams={ 'pattern', 'unsigned int', '7'; 'NSAMP', 'unsigned int', '4*N' }  ClassTemplateParamsEnables={'off', 'off', 'on';'off', 'off', 'on'}  ClassCtorDeclTypeOptions=C[1 1]@t69@polyphase_fir(int16 ( & taps0_i ) [ 64 ], int16 ( & taps1_i ) [ 64 ])  ClassCtorDecl=polyphase_fir(int16 ( & taps0_i ) [ 64 ], int16 ( & taps1_i ) [ 64 ])  ClassCtorParams={ 'taps0_i', 'int16 ( &) [ 64 ]', 'tile7_tapsA'; 'taps1_i', 'int16 ( &) [ 64 ]', 'tile7_tapsB' }  KernelHeaderFile=aie/polyphase_fir.h  KernelClassName=polyphase_fir  KernelFunction=run_i  KernelSourceFile=aie/polyphase_fir.cpp  KernelSearchPaths={}  PreProcOptions={}  blockJsonConstraints=[]
      KernelAllAttrs=|
      | s[12;12;9;9;19;14;21;23;21;23;24;21;15;17;12;24;26;26;26;27;28;9;21;23;23;23;24;25;14;19;19;29]@FunctionNameDeclFileNamePortNamesPortTypesPortSerializedTypesPortDirectionsPortWindowSizeEnablesPortWindowMarginEnablesPortBufferSizeEnablesPortBufferMarginEnablesPortSynchronicityEnablesPortSignalSizeEnablesPortBufferSizesPortBufferMarginsFunctionDeclFunctionTemplateSpecKindFunctionTemplateParamNamesFunctionTemplateParamKindsFunctionTemplateParamTypesFunctionTemplateParamValuesFunctionTemplateParamEnablesClassDeclClassTemplateSpecKindClassTemplateParamNamesClassTemplateParamKindsClassTemplateParamTypesClassTemplateParamValuesClassTemplateParamEnablesClassCtorDeclsClassCtorParamNamesClassCtorParamTypesClassCtorParamSerializedTypes[1 1]@C[32 1]@t5@run_it25@../../aie/polyphase_fir.hC[2 1]@t5@sig_it5@sig_oC[2 1]@t30@input_stream_cint16 * restrictt31@output_stream_cint16 * restrictC[2 1]@t37@{Q2{P{Tinput_stream{1{t{Scint16}}}}}}t38@{Q2{P{Toutput_stream{1{t{Scint16}}}}}}C[2 1]@t5@inputt6@outputC[2 1]@l0@l0@C[2 1]@l0@l0@C[2 1]@l0@l0@C[2 1]@l0@l0@C[2 1]@l0@l0@C[2 1]@l0@l1@C[2 1]@nnC[2 1]@nnt158@template < unsigned int pattern, unsigned int NSAMP > 
      | void polyphase_fir::
      | run_i(input_stream_cint16 * restrict sig_i, output_stream_cint16 * restrict sig_o)t4@nonee[0 1]@e[0 1]@e[0 1]@e[0 1]@e[0 1]@t74@template < unsigned int pattern, unsigned int NSAMP > class polyphase_fir;t8@implicitC[2 1]@t7@patternt5@NSAMPC[2 1]@t7@nontypet7@nontypeC[2 1]@t12@unsigned intt12@unsigned intC[2 1]@nnC[2 1]@l1@l1@C[1 1]@t69@polyphase_fir(int16 ( & taps0_i ) [ 64 ], int16 ( & taps1_i ) [ 64 ])C[1 1]@C[2 1]@t7@taps0_it7@taps1_iC[1 1]@C[2 1]@t17@int16 ( &) [ 64 ]t17@int16 ( &) [ 64 ]C[1 1]@C[2 1]@t14@{R{C{Bi16}64}}t14@{R{C{Bi16}64}}
      FunctionDecl=|
      | template < unsigned int pattern, unsigned int NSAMP > 
      | void polyphase_fir::
      | run_i(input_stream_cint16 * restrict sig_i, output_stream_cint16 * restrict sig_o)
  ChannelizerOut_0 : Outport
  ChannelizerOut_1 : Outport  Port=2
  ChannelizerOut_2 : Outport  Port=3
  ChannelizerOut_3 : Outport  Port=4
  ChannelizerOut_4 : Outport  Port=5
  ChannelizerOut_5 : Outport  Port=6
  ChannelizerOut_6 : Outport  Port=7
  ChannelizerOut_7 : Outport  Port=8
  ToOutputPermute_0 : Outport  Port=9
  ToOutputPermute_1 : Outport  Port=10
  ToOutputPermute_2 : Outport  Port=11
  ToOutputPermute_3 : Outport  Port=12
  ToOutputPermute_4 : Outport  Port=13
  ToOutputPermute_5 : Outport  Port=14
  ToOutputPermute_6 : Outport  Port=15
  ToOutputPermute_7 : Outport  Port=16
  wires:
  PLIO4/1 -> ToOutputPermute_3/1
  PLIO1/1 -> ToOutputPermute_0/1
  PLIO2/1 -> ToOutputPermute_1/1
  PLIO8/1 -> ToOutputPermute_7/1
  PLIO7/1 -> ToOutputPermute_6/1
  PLIO5/1 -> ToOutputPermute_4/1
  PLIO6/1 -> ToOutputPermute_5/1
  PLIO3/1 -> ToOutputPermute_2/1
  PLIO22/1 -> ChannelizerOut_6/1
  PLIO21/1 -> ChannelizerOut_5/1
  PLIO24/1 -> ChannelizerOut_0/1
  PLIO17/1 -> ChannelizerOut_1/1
  PLIO18/1 -> ChannelizerOut_2/1
  PLIO19/1 -> ChannelizerOut_3/1
  PLIO20/1 -> ChannelizerOut_4/1
  PLIO23/1 -> ChannelizerOut_7/1
  run_i1/1 -> PLIO1/1
  run_i7/1 -> PLIO7/1
  run_i6/1 -> PLIO6/1
  PLIO59/1 -> run_i4/1
  PLIO63/1 -> run_i8/1
  FromInputPermute_0/1 -> PLIO48/1
  FromInputPermute_4/1 -> PLIO60/1
  PLIO61/1 -> run_i6/1
  FromInputPermute_2/1 -> PLIO52/1
  PLIO52/1 -> run_i3/1
  FromInputPermute_6/1 -> PLIO62/1
  FromInputPermute_5/1 -> PLIO61/1
  PLIO62/1 -> run_i7/1
  FromInputPermute_3/1 -> PLIO59/1
  run_i5/1 -> PLIO5/1
  FromInputPermute_7/1 -> PLIO63/1
  PLIO49/1 -> run_i2/1
  run_i8/1 -> PLIO8/1
  FromInputPermute_1/1 -> PLIO49/1
  PLIO60/1 -> run_i5/1
  run_i3/1 -> PLIO3/1
  PLIO48/1 -> run_i1/1
  run_i2/1 -> PLIO2/1
  run_i4/1 -> PLIO4/1
  FromCyclicShift_3/1 -> PLIO14/1
  PLIO13/1 -> m16_ssr8_dft_graph/5(y4)
  m16_ssr8_dft_graph/8(u7) -> PLIO23/1
  PLIO16/1 -> m16_ssr8_dft_graph/8(y7)
  FromCyclicShift_5/1 -> PLIO16/1
  m16_ssr8_dft_graph/1(u0) -> PLIO24/1
  FromCyclicShift_2/1 -> PLIO13/1
  m16_ssr8_dft_graph/3(u2) -> PLIO18/1
  FromCyclicShift_1/1 -> PLIO10/1
  m16_ssr8_dft_graph/6(u5) -> PLIO21/1
  m16_ssr8_dft_graph/5(u4) -> PLIO20/1
  PLIO12/1 -> m16_ssr8_dft_graph/4(y3)
  FromCyclicShift_7/1 -> PLIO12/1
  FromCyclicShift_6/1 -> PLIO11/1
  m16_ssr8_dft_graph/2(u1) -> PLIO17/1
  FromCyclicShift_0/1 -> PLIO9/1
  PLIO10/1 -> m16_ssr8_dft_graph/2(y1)
  PLIO11/1 -> m16_ssr8_dft_graph/3(y2)
  PLIO9/1 -> m16_ssr8_dft_graph/1(y0)
  PLIO15/1 -> m16_ssr8_dft_graph/7(y6)
  FromCyclicShift_4/1 -> PLIO15/1
  m16_ssr8_dft_graph/4(u3) -> PLIO19/1
  PLIO14/1 -> m16_ssr8_dft_graph/6(y5)
  m16_ssr8_dft_graph/7(u6) -> PLIO22/1
